simulink model "delay"  (R2020a)
settings: Solver=FixedStepDiscrete  StartTime=0.0  StopTime=inf  RelTol=1e-3
libraries: dspsnks4 x1, dspvision x1
settings Model: Creator=unity  LastModifiedBy=unity
settings SolverCC: AutoInsertRateTranBlk=on
settings DataIOCC: LimitDataPoints=on  SaveOutput=off  SignalLogging=off  SaveTime=off
settings OptimizationCC: LifeSpan=inf
settings DebuggingCC: AlgebraicLoopMsg=error  SingleTaskRateTransMsg=error  AllowSymbolicDim=off  SFUnexpectedBacktrackingDiag=warning  SFNoUnconditionalDefaultTransitionDiag=warning  SFExecutionAtInitializationDiag=none  ArithmeticOperatorsInVariantConditions=warning
settings SFSimCC: SimUseLocalCustomCode=off  CustomCodeUndefinedFunction=UseInterfaceOnly
settings RTWCC: RTWUseLocalCustomCode=off
settings CodeAppCC: StateflowObjectComments=on
settings GRTTargetCC: TargetLangStandard=C89/C90 (ANSI)
settings ConfigComp: CovMetricSettings=dw  CovHtmlReporting=on  CovSaveCumulativeToWorkspaceVar=on  CovSaveSingleToWorkspaceVar=on  CovExternalEMLEnable=off  CovSFcnEnable=off

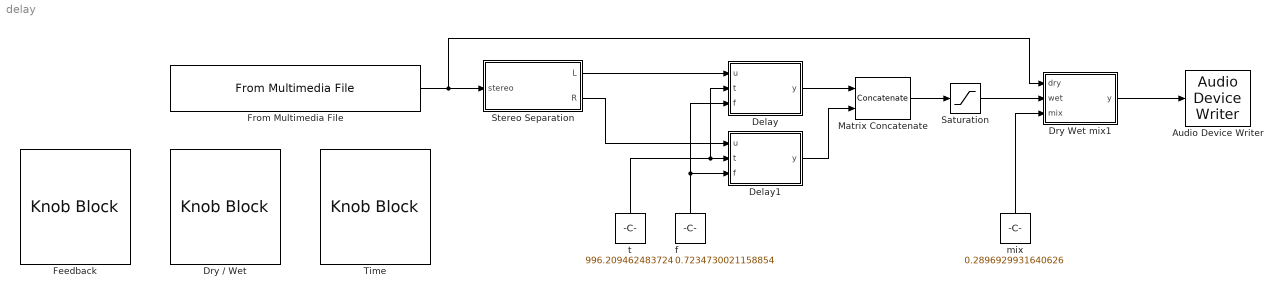
== system delay ==
  Audio Device Writer : dspsnks4/Audio Device Writer  Driver=DirectSound  Device=Default  InheritSampleRate=on  SampleRate=44100  BitDepth=16-bit integer  BufferSize=4096  NumBuffers=10  DefaultOutputChannelMapping=on  OutputChannelMapping=1:2  OutputNumUnderrunSamples=off  DriverIdx=1  DeviceWarnFlag=''
  Delay : MATLAB Function  TreatAsAtomicUnit=on
  Delay1 : MATLAB Function  TreatAsAtomicUnit=on
  Dry / Wet : KnobBlock  ScaleMin=-1  ScaleMax=1
  Dry Wet mix1 : MATLAB Function  TreatAsAtomicUnit=on
  Feedback : KnobBlock  ScaleMax=1
  From Multimedia File : dspvision/From Multimedia File  inputFilename=D:\Program Files\MATLAB\R2020a\toolbox\audio\samples\FunkyDrums-44p1-stereo-25secs.mp3  readRange=[1 Inf]  loop=on  numPlays=inf  outputStreams=オーディオのみ  videoDataType=single  audioDataType=double  inheritSampleTime=on  userDefinedSampleTime=1/30  noAudioOutput=off  isIntensityVideo=off  fourcc=RGB  colorVideoFormat=Separate color signals  outputEOF=off  dataOrg=Column-major  audioFrameSize=256  computeAudioFrameSize=off  outSamplingMode=Sample based
  Matrix Concatenate : Concatenate  Mode=Multidimensional array  ConcatenateDimension=2
  Saturation : Saturate
  Stereo Separation : MATLAB Function  TreatAsAtomicUnit=on
  Time : KnobBlock  ScaleMax=5000
  f : Constant  Value=0.7234730021158854
  mix : Constant  Value=0.2896929931640626
  t : Constant  Tag=a  Value=996.209462483724  OutDataTypeStr=double
  wires:
  From Multimedia File/1 -> Dry Wet mix1/1(dry), Stereo Separation/1(stereo)
  Stereo Separation/1(L) -> Delay/1(u)
  t/1 -> Delay1/2(t), Delay/2(t)
  Stereo Separation/2(R) -> Delay1/1(u)
  f/1 -> Delay1/3(f), Delay/3(f)
  Matrix Concatenate/1 -> Saturation/1
  mix/1 -> Dry Wet mix1/3(mix)
  Delay/1(y) -> Matrix Concatenate/1
  Delay1/1(y) -> Matrix Concatenate/2
  Dry Wet mix1/1(y) -> Audio Device Writer/1
  Saturation/1 -> Dry Wet mix1/2(wet)

== matlab function delay/Delay ==
  data: u input; y output; t input; f input
%パラメータtの追加
function y = fcn(u,t,f)
    %buffer sizeの定義
    buff_size = 100000;

    %frame sizeの定義
    frame_size = length(u);

    %永続変数としてbuffを定義
    persistent buff

    %buffの初期化
    if isempty(buff)
        buff = zeros(buff_size,1);
    end

    %buffをframe_size分動かす
    buff(frame_size+1:buff_size)=buff(1:buff_size-frame_size);

    %現在の入力信号をbuffの先頭に保存
    buff(1:frame_size)=flip(u);
    
    %tサンプル前の音を取り出す
    for index = 1:frame_size
        u(index) = leap(buff,t+index);
    end
    
    u = flip(u);
    
    %フィードバック処理
    buff(1:frame_size) = buff(1:frame_size) + flip(u)*f;

    %出力
        %tサンプル前の音を取り出す
    for index = 1:frame_size
        u(index) = leap(buff,t+index);
    end
    
    u = flip(u);
    
    y = u;

== matlab function delay/Stereo Separation ==
  data: stereo input; L output; R output
function [L,R] = fcn(stereo)
    L = stereo(:,1);
    R = stereo(:,2);

== matlab function delay/Delay1 ==
  data: u input; y output; t input; f input
%パラメータtの追加
function y = fcn(u,t,f)
    %buffer sizeの定義
    buff_size = 100000;

    %frame sizeの定義
    frame_size = length(u);

    %永続変数としてbuffを定義
    persistent buff

    %buffの初期化
    if isempty(buff)
        buff = zeros(buff_size,1);
    end

    %buffをframe_size分動かす
    buff(frame_size+1:buff_size)=buff(1:buff_size-frame_size);

    %現在の入力信号をbuffの先頭に保存
    buff(1:frame_size)=flip(u);
    
    %tサンプル前の音を取り出す
    for index = 1:frame_size
        u(index) = leap(buff,t+index);
    end
    
    u = flip(u);
    
    %フィードバック処理
    buff(1:frame_size) = buff(1:frame_size) + flip(u)*f;

    %出力
        %tサンプル前の音を取り出す
    for index = 1:frame_size
        u(index) = leap(buff,t+index);
    end
    
    u = flip(u);
    
    y = u;

== matlab function delay/Dry Wet mix1 ==
  data: dry input; y output; wet input; mix input
function y = fcn(dry,wet,mix)
    y = dry*min(-mix+1,1)+wet*min(mix+1,1);
